simulink model "AircraftModel_6DoF_Chi"  (R2023b)
settings: Solver=VariableStepAuto  StartTime=0.0  StopTime=20  FixedStep=CNT_StepSize  RelTol=1e-3
values from neighbouring files (symbols this model uses):
  CNT_a = 6378137    [AircraftParameters.m]
  CNT_f = 0.003352810664747    (= 0.00335281066475)    [AircraftParameters.m]
  CNT_g = [0;0;9.81]    [AircraftParameters.m]
  CNT_m = 15975    [AircraftParameters.m]
  ControlLaws =     [ControlLaws.mat]
  Ixx = 102630    [AircraftParameters.m]
  Ixz = 14996    [AircraftParameters.m]
  Iyy = 274335    [AircraftParameters.m]
  Izz = 362250    [AircraftParameters.m]
undefined symbols (not defined in the file or in its folder): Actuators, Aerodynamics, ampl_p_cmd, ARI, beta_cmd, omega_p_cmd, Propulsion, TestSequence, TrimPoint
libraries: simulink x36, vrlib x4, slpidlib x1
(part 2 of 3)

== system AircraftModel_6DoF_Chi/Test Sequences/AoS Test Sequence ==
  Constant : Constant  Value=TrimPoint.States.Altbar
  Constant1 : Constant  Value=sqrt(TrimPoint.States.ubar^2+TrimPoint.States.vbar^2+TrimPoint.States.wbar^2)
  Constant2 : Constant  Value=TrimPoint.States.dabar
  Constant3 : Constant  Value=0
  Gust Generator : Subsystem  mask{gust_start=5, gust_duration=25, gust_amplitude=-30}
      mask prompts: gust_start "start time of the gust in sec"; gust_duration "gust duration in sec"; gust_amplitude "maximum gust speed in m/s"
      mask DialogControl ParameterGroupVar Prompt: gust characteristics
  Step : Step  Time=40  After=beta_cmd  SampleTime=0
  v_Wg : Outport
  u_Wg : Outport  Port=2
  alt_cmd : Outport  Port=3
  cmd_da : Outport  Port=4
  beta_cmd : Outport  Port=5
  V_A_cmd : Outport  Port=6
  wires:
  Constant3/1 -> u_Wg/1  "u_Wg"
  Constant2/1 -> cmd_da/1  "cmd_da"
  Constant1/1 -> V_A_cmd/1  "V_A_cmd"
  Step/1 -> beta_cmd/1  "beta_cmd"
  Constant/1 -> alt_cmd/1  "alt_cmd"
  Gust Generator/1(wind speed) -> v_Wg/1  "v_Wg"

== system AircraftModel_6DoF_Chi/Test Sequences/Bank Angle Test Sequence ==
  Constant : Constant  Value=TrimPoint.States.Altbar
  Constant1 : Constant  Value=sqrt(TrimPoint.States.ubar^2+TrimPoint.States.vbar^2+TrimPoint.States.wbar^2)
  Constant2 : Constant  Value=0
  Constant3 : Constant  Value=0
  Doublet Generator : Subsystem  mask(DoubletGenerator){timeon=5, pulsewidth=20, amplitude=deg2rad(55)}
      mask prompts: timeon "Time Start"; pulsewidth "Pulse Duration"
      mask help:
      | Doublet Generator.
      | Ouputs doublet of specificed amplitude and duration.
      |
      | If start/duration/amplitude parameters are vectors, then output is multichannel.
      mask Display: plot([.1 .3 .3001 .4 .4001 .5  .5001 .7],[0 0 1 1 -1 -1 0 0])
  Gust Generator : Subsystem  mask{gust_start=5, gust_duration=25, gust_amplitude=-30}
      mask prompts: gust_start "start time of the gust in sec"; gust_duration "gust duration in sec"; gust_amplitude "maximum gust speed in m/s"
      mask DialogControl ParameterGroupVar Prompt: gust characteristics
  v_Wg : Outport
  u_Wg : Outport  Port=2
  alt_cmd : Outport  Port=3
  Phi_cmd : Outport  Port=4
  beta_cmd : Outport  Port=5
  V_A_cmd : Outport  Port=6
  wires:
  Constant3/1 -> u_Wg/1  "u_Wg"
  Doublet Generator/1(Doublet) -> Phi_cmd/1  "Phi_cmd"
  Constant1/1 -> V_A_cmd/1  "V_A_cmd"
  Constant2/1 -> beta_cmd/1  "beta_cmd"
  Constant/1 -> alt_cmd/1  "alt_cmd"
  Gust Generator/1(wind speed) -> v_Wg/1  "v_Wg"

== system AircraftModel_6DoF_Chi/Test Sequences/Course Angle Test Sequence ==
  Constant : Constant  Value=TrimPoint.States.Altbar
  Constant1 : Constant  Value=sqrt(TrimPoint.States.ubar^2+TrimPoint.States.vbar^2+TrimPoint.States.wbar^2)
  Constant2 : Constant  Value=0
  Constant3 : Constant  Value=0
  Gust Generator : Subsystem  mask{gust_start=40, gust_duration=25, gust_amplitude=-30}
      mask prompts: gust_start "start time of the gust in sec"; gust_duration "gust duration in sec"; gust_amplitude "maximum gust speed in m/s"
      mask DialogControl ParameterGroupVar Prompt: gust characteristics
  Step1 : Step  Time=10  Before=TrimPoint.States.Psibar  After=deg2rad(350)  SampleTime=0
  v_Wg : Outport
  u_Wg : Outport  Port=2
  alt_cmd : Outport  Port=3
  Chi_cmd : Outport  Port=4
  beta_cmd : Outport  Port=5
  V_A_cmd : Outport  Port=6
  wires:
  Constant3/1 -> u_Wg/1  "u_Wg"
  Step1/1 -> Chi_cmd/1  "Chi_cmd"
  Constant1/1 -> V_A_cmd/1  "V_A_cmd"
  Constant2/1 -> beta_cmd/1  "beta_cmd"
  Constant/1 -> alt_cmd/1  "alt_cmd"
  Gust Generator/1(wind speed) -> v_Wg/1  "v_Wg"

== system AircraftModel_6DoF_Chi/Test Sequences/Default ==
  Constant : Constant  Value=TrimPoint.States.Altbar
  Constant1 : Constant  Value=sqrt(TrimPoint.States.ubar^2+TrimPoint.States.vbar^2+TrimPoint.States.wbar^2)
  Constant2 : Constant  Value=TrimPoint.States.dabar
  Constant3 : Constant  Value=0
  Constant4 : Constant  Value=TrimPoint.States.drbar
  Constant5 : Constant  Value=0
  v_Wg : Outport
  u_Wg : Outport  Port=2
  alt_cmd : Outport  Port=3
  cmd_da : Outport  Port=4
  cmd_dr : Outport  Port=5
  V_A_cmd : Outport  Port=6
  wires:
  Constant/1 -> alt_cmd/1  "alt_cmd"
  Constant1/1 -> V_A_cmd/1  "V_A_cmd"
  Constant2/1 -> cmd_da/1  "cmd_da"
  Constant4/1 -> cmd_dr/1  "cmd_dr"
  Constant5/1 -> v_Wg/1  "v_Wg"
  Constant3/1 -> u_Wg/1  "u_Wg"

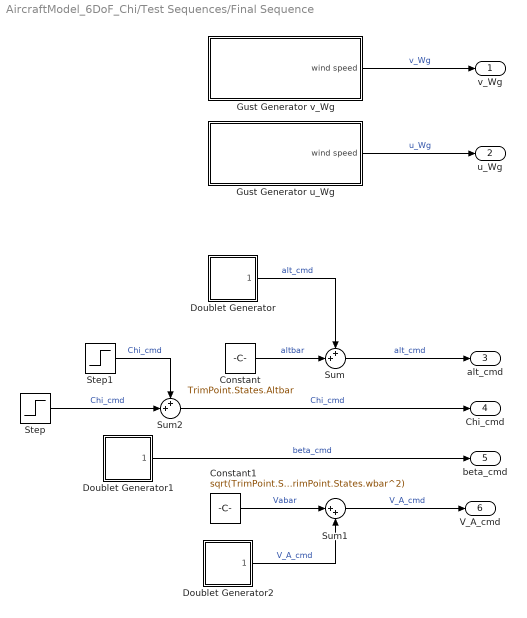
== system AircraftModel_6DoF_Chi/Test Sequences/Final Sequence ==
  Constant : Constant  Value=TrimPoint.States.Altbar
  Constant1 : Constant  Value=sqrt(TrimPoint.States.ubar^2+TrimPoint.States.vbar^2+TrimPoint.States.wbar^2)
  Doublet Generator : Subsystem  mask(DoubletGenerator){timeon=15, pulsewidth=40, amplitude=200}
      mask prompts: timeon "Time Start"; pulsewidth "Pulse Duration"
      mask help:
      | Doublet Generator.
      | Ouputs doublet of specificed amplitude and duration.
      |
      | If start/duration/amplitude parameters are vectors, then output is multichannel.
      mask Display: plot([.1 .3 .3001 .4 .4001 .5  .5001 .7],[0 0 1 1 -1 -1 0 0])
  Doublet Generator1 : Subsystem  mask(DoubletGenerator){timeon=60, pulsewidth=20, amplitude=deg2rad(3)}
      mask prompts: timeon "Time Start"; pulsewidth "Pulse Duration"
      mask help:
      | Doublet Generator.
      | Ouputs doublet of specificed amplitude and duration.
      |
      | If start/duration/amplitude parameters are vectors, then output is multichannel.
      mask Display: plot([.1 .3 .3001 .4 .4001 .5  .5001 .7],[0 0 1 1 -1 -1 0 0])
  Doublet Generator2 : Subsystem  mask(DoubletGenerator){timeon=10, pulsewidth=40, amplitude=-20}
      mask prompts: timeon "Time Start"; pulsewidth "Pulse Duration"
      mask help:
      | Doublet Generator.
      | Ouputs doublet of specificed amplitude and duration.
      |
      | If start/duration/amplitude parameters are vectors, then output is multichannel.
      mask Display: plot([.1 .3 .3001 .4 .4001 .5  .5001 .7],[0 0 1 1 -1 -1 0 0])
  Gust Generator u_Wg : Subsystem  mask{gust_start=60, gust_duration=15, gust_amplitude=-30}
      mask prompts: gust_start "start time of the gust in sec"; gust_duration "gust duration in sec"; gust_amplitude "maximum gust speed in m/s"
      mask DialogControl ParameterGroupVar Prompt: gust characteristics
  Gust Generator v_Wg : Subsystem  mask{gust_start=20, gust_duration=25, gust_amplitude=-30}
      mask prompts: gust_start "start time of the gust in sec"; gust_duration "gust duration in sec"; gust_amplitude "maximum gust speed in m/s"
      mask DialogControl ParameterGroupVar Prompt: gust characteristics
  Step : Step  Time=10  Before=TrimPoint.States.Psibar  After=deg2rad(10)  SampleTime=0
  Step1 : Step  Time=80  After=deg2rad(170)  SampleTime=0
  Sum : Sum  Inputs=++|
  Sum1 : Sum  Inputs=|++
  Sum2 : Sum  Inputs=++|
  v_Wg : Outport
  u_Wg : Outport  Port=2
  alt_cmd : Outport  Port=3
  Chi_cmd : Outport  Port=4
  beta_cmd : Outport  Port=5
  V_A_cmd : Outport  Port=6
  wires:
  Sum2/1 -> Chi_cmd/1  "Chi_cmd"
  Gust Generator u_Wg/1(wind speed) -> u_Wg/1  "u_Wg"
  Step1/1 -> Sum2/1  "Chi_cmd"
  Constant1/1 -> Sum1/1  "Vabar"
  Step/1 -> Sum2/2  "Chi_cmd"
  Doublet Generator/1(Doublet) -> Sum/1  "alt_cmd"
  Sum/1 -> alt_cmd/1  "alt_cmd"
  Gust Generator v_Wg/1(wind speed) -> v_Wg/1  "v_Wg"
  Doublet Generator2/1(Doublet) -> Sum1/2  "V_A_cmd"
  Constant/1 -> Sum/2  "altbar"
  Doublet Generator1/1(Doublet) -> beta_cmd/1  "beta_cmd"
  Sum1/1 -> V_A_cmd/1  "V_A_cmd"

== system AircraftModel_6DoF_Chi/Test Sequences/Roll Rate Test Sequence ==
  Constant : Constant  Value=TrimPoint.States.Altbar
  Constant1 : Constant  Value=sqrt(TrimPoint.States.ubar^2+TrimPoint.States.vbar^2+TrimPoint.States.wbar^2)
  Constant2 : Constant  Value=0
  Constant3 : Constant  Value=0
  Constant4 : Constant  Value=0
  Sine Wave1 : Sin  Amplitude=ampl_p_cmd  Frequency=omega_p_cmd  SampleTime=0
  v_Wg : Outport
  u_Wg : Outport  Port=2
  alt_cmd : Outport  Port=3
  p_cmd : Outport  Port=4
  beta_cmd : Outport  Port=5
  V_A_cmd : Outport  Port=6
  wires:
  Constant3/1 -> u_Wg/1  "u_Wg"
  Constant1/1 -> V_A_cmd/1  "V_A_cmd"
  Constant2/1 -> beta_cmd/1  "beta_cmd"
  Constant/1 -> alt_cmd/1  "alt_cmd"
  Constant4/1 -> v_Wg/1  "v_Wg"
  Sine Wave1/1 -> p_cmd/1  "p_cmd"

== system AircraftModel_6DoF_Chi/Test Sequences/SAS Test Sequence ==
  Constant : Constant  Value=TrimPoint.States.Altbar
  Constant1 : Constant  Value=sqrt(TrimPoint.States.ubar^2+TrimPoint.States.vbar^2+TrimPoint.States.wbar^2)
  Constant2 : Constant  Value=TrimPoint.States.dabar
  Constant3 : Constant  Value=0
  Gust Generator : Subsystem  mask{gust_start=5, gust_duration=25, gust_amplitude=-30}
      mask prompts: gust_start "start time of the gust in sec"; gust_duration "gust duration in sec"; gust_amplitude "maximum gust speed in m/s"
      mask DialogControl ParameterGroupVar Prompt: gust characteristics
  Step : Step  Time=40  After=deg2rad(5)  SampleTime=0
  v_Wg : Outport
  u_Wg : Outport  Port=2
  alt_cmd : Outport  Port=3
  cmd_da : Outport  Port=4
  cmd_dr : Outport  Port=5
  V_A_cmd : Outport  Port=6
  wires:
  Constant/1 -> alt_cmd/1  "alt_cmd"
  Constant1/1 -> V_A_cmd/1  "V_A_cmd"
  Constant2/1 -> cmd_da/1  "cmd_da"
  Step/1 -> cmd_dr/1  "cmd_dr"
  Gust Generator/1(wind speed) -> v_Wg/1  "v_Wg"
  Constant3/1 -> u_Wg/1  "u_Wg"

== system AircraftModel_6DoF_Chi/Equations of Motion/Calculation of Position_dot/ZeroOffset - cos (Lat) ==
  In : Inport
  Abs : Abs
  Constant : Constant  Value=tol  SampleTime=-1
  Non-zero Sign : Subsystem  mask(Non-zero sign){}
      mask help: Sign function outputs 1 for input greater than or equal to 0, and -1 otherwise.
  Product : Product  InputSameDT=on  SaturateOnIntegerOverflow=on  OutDataTypeStr=Inherit: Same as first input
  Switch : Switch  Threshold=tol
  Out : Outport
  wires:
  In/1 -> Switch/1, Non-zero Sign/1(In), Abs/1
  Abs/1 -> Switch/2
  Non-zero Sign/1(Out) -> Product/1
  Constant/1 -> Product/2
  Product/1 -> Switch/3
  Switch/1 -> Out/1

== system AircraftModel_6DoF_Chi/Flight Controls/Lateral Directional Control Laws/Aileron Rudder Interconnection ==
  cmd_da_in : Inport
  cmd_dr_in : Inport  Port=2
  ARI : Constant  Value=ARI
  Demux : Demux  Outputs=2
  Mux : Mux  Inputs=2
  Product : Product  Multiplication=Matrix(*)
  cmd_da_ARI : Outport
  cmd_dr_ARI : Outport  Port=2
  wires:
  cmd_da_in/1 -> Mux/1
  ARI/1 -> Product/1
  Demux/1 -> cmd_da_ARI/1
  Demux/2 -> cmd_dr_ARI/1
  Product/1 -> Demux/1
  cmd_dr_in/1 -> Mux/2
  Mux/1 -> Product/2

== system AircraftModel_6DoF_Chi/Flight Controls/Lateral Directional Control Laws/Bank Angle Control ==
  note: Proportional
      | Gain
  In1 : Inport
  Gain5 : Gain  Gain=ControlLaws.LatDirMot.BankAngle.Kp
  Saturation : Saturate  UpperLimit=12.5  LowerLimit=-12.5
  Out1 : Outport
  wires:
  Gain5/1 -> Saturation/1
  In1/1 -> Gain5/1
  Saturation/1 -> Out1/1

== system AircraftModel_6DoF_Chi/Flight Controls/Lateral Directional Control Laws/Course Angle Controller ==
  note: Proportional
      | Gain
  In1 : Inport
  Gain5 : Gain  Gain=ControlLaws.LatDirMot.Course.Kp
  Saturation : Saturate  UpperLimit=40  LowerLimit=-40
  Out1 : Outport
  wires:
  In1/1 -> Gain5/1
  Gain5/1 -> Saturation/1
  Saturation/1 -> Out1/1

== system AircraftModel_6DoF_Chi/Flight Controls/Lateral Directional Control Laws/Roll Rate Control ==
  note: Integrator Boost
  note: Lead/Lag Compensator
  note: Proportional
      | Gain
  note: Roll-Off Compensator
  In1 : Inport
  Input : Inport  Port=2
  Cond. Int. Anti Windup : Subsystem  mask(Integrator Anti-Windup){max_u=inf, min_u=-inf, negative_sign=off}
      mask prompts: max_u "Maximum control signal"; min_u "Minimum control signal"; negative_sign "Negative amplification in control law"
      mask help:
      | This block provides integration using the "conditional integration" anti-windup compensation.
      | It compares the sign of the error and the sign of the control signal and stops integration in case the error drives saturation.
      mask Help:
      | This block provides integration using the "conditional integration" anti-windup compensation. It stops or continues integration depending on the sign of the integrator input (control error) and the commanded control signal. Only if the input would further increase the already saturated integrator output, integration is stopped. This method is different from "integrator clamping" and and "integrator back calculation" and usually provides better recovery properties.
      | 
      | In a standard control architecture the inputs are as follows:
      | INPUT is the error signal r-y
      | RESET is a reset signal. The integrator state is reseted on either rising or falling edges
      | X0 is the initial condition for the integrator
      | U is the commanded control signal
      | 
      | For the anti-windup to work as intended, a saturation block must be placed on the ouput of the control command being fed to the associated actuator, which should include all control signal contributions (e.g. from proportional feedback and inner loops). U is the signal before this saturation.
      | 
      | The default logic assumes a plant with positive steady-state gain to be controlled. This translates to the following logic:
      | For commanded control signal u, saturation limits Umax and Umin, and error e,
      | If u is in bounds, do nothing
      | If u >= Umax AND e > 0, stop integrating
      | If u >= Umax AND e < 0, continue integrating
      | If u <= Umin AND e > 0, continue integrating
      | If u <= Umin AND e < 0, stop integrating
      | 
      | If a plant with negative steady-state gain is to be controlled (e.g. pitch), the windup logic may changed using the NEGATIVE SIGN option. (Note: If unsure check if the controller gains are negative. If yes, check the NEGATIVE SIGN option)
      | This then translates to the logic:
      | If u is in bounds, do nothing
      | If u >= Umax AND e < 0, stop integrating
      | If u >= Umax AND e > 0, continue integrating
      | If u <= Umin AND e < 0, continue integrating
      | If u <= Umin AND e > 0, stop integrating
  Gain3 : Gain  Gain=ControlLaws.LatDirMot.RollRate.Klz
  Gain4 : Gain  Gain=ControlLaws.LatDirMot.RollRate.Klp
  Gain5 : Gain  Gain=ControlLaws.LatDirMot.RollRate.Kp
  Gain6 : Gain  Gain=ControlLaws.LatDirMot.RollRate.Kr
  Gain7 : Gain  Gain=ControlLaws.LatDirMot.RollRate.Ki
  Integrator2 : Integrator  UpperSaturationLimit=max(Actuators.Limits.u_max_He)  LowerSaturationLimit=min(Actuators.Limits.u_max_He)  ContinuousStateAttributes='K'
  Integrator3 : Integrator  UpperSaturationLimit=max(Actuators.Limits.u_max_He)  LowerSaturationLimit=min(Actuators.Limits.u_max_He)  ContinuousStateAttributes='K'
  Integrator4 : Integrator  UpperSaturationLimit=max(Actuators.Limits.u_max_He)  LowerSaturationLimit=min(Actuators.Limits.u_max_He)  ContinuousStateAttributes='K'
  Integrator5 : Integrator  InitialCondition=TrimPoint.States.dabar  UpperSaturationLimit=max(Actuators.Limits.u_max_He)  LowerSaturationLimit=min(Actuators.Limits.u_max_He)  ContinuousStateAttributes='K'
  Saturation : Saturate  UpperLimit=max(Actuators.Limits.u_max_Hr)  LowerLimit=max(Actuators.Limits.u_max_Hr)
  Sum1 : Sum  Inputs=|++
  Sum3 : Sum  Inputs=|+-
  Sum6 : Sum  Inputs=|+-
  Sum7 : Sum  Inputs=|++
  cmd_da_in : Outport
  wires:
  Sum7/1 -> Saturation/1
  Integrator5/1 -> Sum7/1
  Gain5/1 -> Sum6/1
  Input/1 -> Cond. Int. Anti Windup/2(u)
  Gain7/1 -> Cond. Int. Anti Windup/1(in)
  Sum3/1 -> Gain7/1, Sum7/2, Gain4/1
  Gain6/1 -> Integrator4/1
  Cond. Int. Anti Windup/1(out) -> Integrator5/1
  Sum6/1 -> Gain6/1
  Saturation/1 -> cmd_da_in/1
  Gain4/1 -> Integrator3/1
  Integrator2/1 -> Sum1/1
  Sum1/1 -> Sum3/1
  Integrator3/1 -> Sum3/2
  Gain3/1 -> Integrator2/1
  Integrator4/1 -> Sum6/2, Sum1/2, Gain3/1
  In1/1 -> Gain5/1

== system AircraftModel_6DoF_Chi/Flight Controls/Lateral Directional Control Laws/Sideslip Angle Control ==
  note: Proportional
      | Gain
  note: Roll-Off Compensator
  note: Lead/Lag Compensator
  note: Integrator Boost
  In1 : Inport
  Input : Inport  Port=2
  Cond. Int. Anti Windup : Subsystem  mask(Integrator Anti-Windup){max_u=inf, min_u=-inf, negative_sign=off}
      mask prompts: max_u "Maximum control signal"; min_u "Minimum control signal"; negative_sign "Negative amplification in control law"
      mask help:
      | This block provides integration using the "conditional integration" anti-windup compensation.
      | It compares the sign of the error and the sign of the control signal and stops integration in case the error drives saturation.
      mask Help:
      | This block provides integration using the "conditional integration" anti-windup compensation. It stops or continues integration depending on the sign of the integrator input (control error) and the commanded control signal. Only if the input would further increase the already saturated integrator output, integration is stopped. This method is different from "integrator clamping" and and "integrator back calculation" and usually provides better recovery properties.
      | 
      | In a standard control architecture the inputs are as follows:
      | INPUT is the error signal r-y
      | RESET is a reset signal. The integrator state is reseted on either rising or falling edges
      | X0 is the initial condition for the integrator
      | U is the commanded control signal
      | 
      | For the anti-windup to work as intended, a saturation block must be placed on the ouput of the control command being fed to the associated actuator, which should include all control signal contributions (e.g. from proportional feedback and inner loops). U is the signal before this saturation.
      | 
      | The default logic assumes a plant with positive steady-state gain to be controlled. This translates to the following logic:
      | For commanded control signal u, saturation limits Umax and Umin, and error e,
      | If u is in bounds, do nothing
      | If u >= Umax AND e > 0, stop integrating
      | If u >= Umax AND e < 0, continue integrating
      | If u <= Umin AND e > 0, continue integrating
      | If u <= Umin AND e < 0, stop integrating
      | 
      | If a plant with negative steady-state gain is to be controlled (e.g. pitch), the windup logic may changed using the NEGATIVE SIGN option. (Note: If unsure check if the controller gains are negative. If yes, check the NEGATIVE SIGN option)
      | This then translates to the logic:
      | If u is in bounds, do nothing
      | If u >= Umax AND e < 0, stop integrating
      | If u >= Umax AND e > 0, continue integrating
      | If u <= Umin AND e < 0, continue integrating
      | If u <= Umin AND e > 0, stop integrating
  Gain3 : Gain  Gain=ControlLaws.LatDirMot.AoS.Klz
  Gain4 : Gain  Gain=ControlLaws.LatDirMot.AoS.Klp
  Gain5 : Gain  Gain=ControlLaws.LatDirMot.AoS.Kp
  Gain6 : Gain  Gain=ControlLaws.LatDirMot.AoS.Kr
  Gain7 : Gain  Gain=ControlLaws.LatDirMot.AoS.Ki
  Integrator2 : Integrator  UpperSaturationLimit=max(Actuators.Limits.u_max_He)  LowerSaturationLimit=min(Actuators.Limits.u_max_He)  ContinuousStateAttributes='K'
  Integrator3 : Integrator  UpperSaturationLimit=max(Actuators.Limits.u_max_He)  LowerSaturationLimit=min(Actuators.Limits.u_max_He)  ContinuousStateAttributes='K'
  Integrator4 : Integrator  UpperSaturationLimit=max(Actuators.Limits.u_max_He)  LowerSaturationLimit=min(Actuators.Limits.u_max_He)  ContinuousStateAttributes='K'
  Integrator5 : Integrator  InitialCondition=TrimPoint.States.drbar  UpperSaturationLimit=max(Actuators.Limits.u_max_He)  LowerSaturationLimit=min(Actuators.Limits.u_max_He)  ContinuousStateAttributes='K'
  Saturation : Saturate  UpperLimit=max(Actuators.Limits.u_max_Hr)  LowerLimit=max(Actuators.Limits.u_max_Hr)
  Sum1 : Sum  Inputs=|++
  Sum3 : Sum  Inputs=|+-
  Sum6 : Sum  Inputs=|+-
  Sum7 : Sum  Inputs=|++
  cmd_dr_in : Outport
  wires:
  In1/1 -> Gain5/1
  Saturation/1 -> cmd_dr_in/1
  Gain5/1 -> Sum6/1
  Sum6/1 -> Gain6/1
  Gain6/1 -> Integrator4/1
  Integrator4/1 -> Sum6/2, Sum1/2, Gain3/1
  Integrator3/1 -> Sum3/2
  Gain3/1 -> Integrator2/1
  Sum1/1 -> Sum3/1
  Gain4/1 -> Integrator3/1
  Integrator2/1 -> Sum1/1
  Sum7/1 -> Saturation/1
  Sum3/1 -> Gain7/1, Sum7/2, Gain4/1
  Integrator5/1 -> Sum7/1
  Gain7/1 -> Cond. Int. Anti Windup/1(in)
  Input/1 -> Cond. Int. Anti Windup/2(u)
  Cond. Int. Anti Windup/1(out) -> Integrator5/1

== system AircraftModel_6DoF_Chi/Flight Controls/Lateral Directional Control Laws/yaw damper ==
  note: LowPass Filter
  note: Proportional
      | Gain
  r : Inport
  Gain1 : Gain  Gain=ControlLaws.LatDirMot.SAS.omega_lp
  Gain5 : Gain  Gain=ControlLaws.LatDirMot.SAS.kr
  Integrator1 : Integrator  UpperSaturationLimit=max(Actuators.Limits.u_max_He)  LowerSaturationLimit=min(Actuators.Limits.u_max_He)  ContinuousStateAttributes='K'
  Sum2 : Sum  Inputs=|+-
  Washout Filter : Subsystem  mask{wb=ControlLaws.LatDirMot.SAS.omega_wo}
      mask prompts: wb "Filter Bandwidth"
      mask Display:
      | plot([0.35 0.5 0.65 ],[0.4 0.6 0.6 ]);
      | text(0.5,0.3,[num2str(wb) ' rad/s'],'horizontalAlignment', 'center');
      | text(0.67,0.6,['1'],'horizontalAlignment', 'left');
  dr : Outport
  wires:
  r/1 -> Washout Filter/1(Input)
  Sum2/1 -> Integrator1/1
  Gain1/1 -> Sum2/2
  Integrator1/1 -> Gain1/1, Gain5/1
  Washout Filter/1(Output) -> Sum2/1  "cmd_dr"
  Gain5/1 -> dr/1

== system AircraftModel_6DoF_Chi/Flight Controls/Longitudinal Control Laws/Subsystem ==
  Theta : Inport
  uf : Inport  Port=2
  wf : Inport  Port=3
  Cos : Trigonometry  Operator=cos
  Product : Product
  Product1 : Product
  Sin : Trigonometry
  Sum : Sum  Inputs=|+-
  hdot : Outport
  wires:
  Sum/1 -> hdot/1
  Product1/1 -> Sum/2
  Product/1 -> Sum/1
  Cos/1 -> Product1/1
  wf/1 -> Product1/2
  uf/1 -> Product/2
  Sin/1 -> Product/1
  Theta/1 -> Sin/1, Cos/1

== system AircraftModel_6DoF_Chi/Flight Controls/Longitudinal Control Laws/alt_control ==
  In1 : Inport
  Gain3 : Gain  Gain=ControlLaws.LonMot.Altitude.Klp
  Gain4 : Gain  Gain=10*ControlLaws.LonMot.Altitude.Klz
  Gain5 : Gain  Gain=ControlLaws.LonMot.Altitude.Kp
  Gain6 : Gain  Gain=ControlLaws.LonMot.Altitude.Kr
  Integrator2 : Integrator  UpperSaturationLimit=max(Actuators.Limits.u_max_He)  LowerSaturationLimit=min(Actuators.Limits.u_max_He)  ContinuousStateAttributes='Khdot'
  Integrator3 : Integrator  UpperSaturationLimit=max(Actuators.Limits.u_max_He)  LowerSaturationLimit=min(Actuators.Limits.u_max_He)  ContinuousStateAttributes='K'
  Integrator4 : Integrator  UpperSaturationLimit=max(Actuators.Limits.u_max_He)  LowerSaturationLimit=min(Actuators.Limits.u_max_He)  ContinuousStateAttributes='Khdot'
  Saturation2 : Saturate  UpperLimit=ControlLaws.Saturations.hdot(2)  LowerLimit=ControlLaws.Saturations.hdot(1)
  Sum1 : Sum  Inputs=|++
  Sum3 : Sum  Inputs=|+-
  Sum6 : Sum  Inputs=|+-
  Out1 : Outport
  wires:
  In1/1 -> Gain5/1
  Sum3/1 -> Sum6/1, Gain4/1
  Gain5/1 -> Gain3/1, Sum1/2
  Integrator4/1 -> Sum6/2, Saturation2/1
  Saturation2/1 -> Out1/1
  Integrator2/1 -> Sum1/1
  Sum1/1 -> Sum3/1
  Gain4/1 -> Integrator3/1
  Integrator3/1 -> Sum3/2
  Gain3/1 -> Integrator2/1
  Sum6/1 -> Gain6/1
  Gain6/1 -> Integrator4/1

== system AircraftModel_6DoF_Chi/Flight Controls/Longitudinal Control Laws/athrl_control ==
  In1 : Inport
  Gain2 : Gain  Gain=ControlLaws.LonMot.ATHR.Kr
  Gain3 : Gain  Gain=-ControlLaws.LonMot.ATHR.Kp
  Gain4 : Gain  Gain=ControlLaws.LonMot.ATHR.Klp
  Gain8 : Gain  Gain=ControlLaws.LonMot.ATHR.Klz
  Integrator1 : Integrator  UpperSaturationLimit=max(Actuators.Limits.u_max_He)  LowerSaturationLimit=min(Actuators.Limits.u_max_He)  ContinuousStateAttributes='K'
  Integrator2 : Integrator  UpperSaturationLimit=max(Actuators.Limits.u_max_He)  LowerSaturationLimit=min(Actuators.Limits.u_max_He)  ContinuousStateAttributes='K'
  Integrator3 : Integrator  UpperSaturationLimit=max(Actuators.Limits.u_max_He)  LowerSaturationLimit=min(Actuators.Limits.u_max_He)  ContinuousStateAttributes='K'
  Sum2 : Sum  Inputs=|+-
  Sum3 : Sum  Inputs=|++
  Sum4 : Sum  Inputs=|+-
  Out1 : Outport
  wires:
  Integrator2/1 -> Sum3/1
  Integrator3/1 -> Sum4/2
  Gain3/1 -> Gain4/1, Sum3/2
  In1/1 -> Gain3/1
  Sum3/1 -> Sum4/1
  Integrator1/1 -> Sum2/2, Out1/1
  Gain2/1 -> Integrator1/1
  Sum2/1 -> Gain2/1
  Gain4/1 -> Integrator2/1
  Gain8/1 -> Integrator3/1
  Sum4/1 -> Gain8/1, Sum2/1

== system AircraftModel_6DoF_Chi/Flight Controls/Longitudinal Control Laws/hdot_control ==
  In1 : Inport
  Gain3 : Gain  Gain=0.1*ControlLaws.LonMot.ClimbRate.Klp
  Gain4 : Gain  Gain=10*ControlLaws.LonMot.ClimbRate.Klz
  Gain5 : Gain  Gain="1.8  %ControlLaws.LonMot.ClimbRate.Kp"
  Gain6 : Gain  Gain=ControlLaws.LonMot.ClimbRate.Kr
  Integrator2 : Integrator  UpperSaturationLimit=max(Actuators.Limits.u_max_He)  LowerSaturationLimit=min(Actuators.Limits.u_max_He)  ContinuousStateAttributes='Khdot'
  Integrator3 : Integrator  UpperSaturationLimit=max(Actuators.Limits.u_max_He)  LowerSaturationLimit=min(Actuators.Limits.u_max_He)  ContinuousStateAttributes='K'
  Integrator4 : Integrator  UpperSaturationLimit=max(Actuators.Limits.u_max_He)  LowerSaturationLimit=min(Actuators.Limits.u_max_He)  ContinuousStateAttributes='Khdot'
  PID Controller : slpidlib/PID Controller  Controller=I  Form=Parallel  TimeDomain=Continuous-time  UseExternalTs=off  SampleTime=-1  IntegratorMethod=Forward Euler  FilterMethod=Forward Euler  ControllerParametersSource=internal  P=1.2  I=0.45  UseKiTs=off  D=1  N=100  UseFilter=on  TunerSelectOption=Transfer Function Based (PID Tuner App)  InitialConditionSource=internal  InitialConditionForIntegrator=0  InitialConditionForFilter=0  DifferentiatorICPrevScaledInput=0  ExternalReset=none  TrackingMode=off  Kt=1  LimitOutput=off  SatLimitsSource=internal  UpperSaturationLimit=inf  LowerSaturationLimit=-inf  LinearizeAsGain=on  AntiWindupMode=none  Kb=1  LimitIntegrator=off  UpperIntegratorSaturationLimit=inf  LowerIntegratorSaturationLimit=-inf  POutMin=[]  POutMax=[]  IOutMin=[]  IOutMax=[]  DOutMin=[]  DOutMax=[]  NOutMin=[]  NOutMax=[]  SumOutMin=[]  SumOutMax=[]  SaturationOutMin=[]  SaturationOutMax=[]  PParamMin=[]  PParamMax=[]  IParamMin=[]  IParamMax=[]  DParamMin=[]  DParamMax=[]  NParamMin=[]  NParamMax=[]  KbParamMin=[]  KbParamMax=[]  KtParamMin=[]  KtParamMax=[]  KbOutMin=[]  KbOutMax=[]  KtOutMin=[]  KtOutMax=[]  IntegratorOutMin=[]  IntegratorOutMax=[]  FilterOutMin=[]  FilterOutMax=[]  SumI1OutMin=[]  SumI1OutMax=[]  SumI2OutMin=[]  SumI2OutMax=[]  SumI3OutMin=[]  SumI3OutMax=[]  SumI4OutMin=[]  SumI4OutMax=[]  SumDOutMin=[]  SumDOutMax=[]  DifferentiatorOutMin=[]  DifferentiatorOutMax=[]  FilterDiffOutCoefMin=[]  FilterDiffOutCoefMax=[]  ReciprocalOutMin=[]  ReciprocalOutMax=[]  SumDenOutMin=[]  SumDenOutMax=[]  SumNumOutMin=[]  SumNumOutMax=[]  DivideOutMin=[]  DivideOutMax=[]  UdiffTsProdOutMin=[]  UdiffTsProdOutMax=[]  NTsProdOutMin=[]  NTsProdOutMax=[]  UintegralTsProdOutMin=[]  UintegralTsProdOutMax=[]  UngainTsProdOutMin=[]  UngainTsProdOutMax=[]  ClampingZeroOutDataTypeStr=Inherit: Inherit via back propagation  ClampingZeroOutMin=[]  ClampingZeroOutMax=[]  FilterDenConstantOutDataTypeStr=Inherit: Inherit via back propagation  FilterDenConstantOutMin=[]  FilterDenConstantOutMax=[]  PCopyOutDataTypeStr=Inherit: Inherit via back propagation  PCopyOutMin=[]  PCopyOutMax=[]  NCopyOutDataTypeStr=Inherit: Inherit via back propagation  NCopyOutMin=[]  NCopyOutMax=[]  IntegratorContinuousStateAttributes=''  IntegratorStateMustResolveToSignalObject=off  IntegratorRTWStateStorageClass=Auto  FilterContinuousStateAttributes=''  FilterStateMustResolveToSignalObject=off  FilterRTWStateStorageClass=Auto  ParallelPVariant=Disabled  IdealPVariant=Disabled  IVariant=InternalParameters  DVariant=Disabled  IntegratorVariant=Continuous  SatVariant=Disabled  AWVariant=Passthrough  PCopyVariant=Disabled  TRVariant=Disabled  FdbkBlocksVariant=Forward  IdealPFdbkVariant=Disabled  SatFdbkVariant=Disabled  DerivativeFilterVariant=Disabled  NVariant=Disabled  NCopyVariant=Disabled_SignalSpec  FilterICVariant=Disabled  IntegratorICVariant=InternalICs  ExternalResetVariant=Disabled  TRSumVariant=Passthrough  SumFdbkVariant=Disabled  SumVariant=Passthrough_I  TsampFilterVariant=InternalTs  TsampNgainVariant=Passthrough  TsampIntegralVariant=Disabled_SignalSpec  ExternalSaturationOutDataTypeStr=Inherit: Same as second input
  Saturation2 : Saturate  UpperLimit=ControlLaws.Saturations.nz(2)  LowerLimit=ControlLaws.Saturations.nz(1)
  Sum1 : Sum  Inputs=|++
  Sum3 : Sum  Inputs=|+-
  Sum6 : Sum  Inputs=|+-
  Out1 : Outport
  wires:
  PID Controller/1 -> Saturation2/1
  In1/1 -> Gain5/1
  Sum3/1 -> Sum6/1, Gain4/1
  Gain5/1 -> Gain3/1, Sum1/2
  Integrator4/1 -> Sum6/2, PID Controller/1
  Saturation2/1 -> Out1/1
  Integrator2/1 -> Sum1/1
  Sum1/1 -> Sum3/1
  Gain4/1 -> Integrator3/1
  Integrator3/1 -> Sum3/2
  Gain3/1 -> Integrator2/1
  Sum6/1 -> Gain6/1
  Gain6/1 -> Integrator4/1

== system AircraftModel_6DoF_Chi/Flight Controls/Longitudinal Control Laws/nz_control ==
  In1 : Inport
  Inport : Inport  Port=2
  Cond. Int. Anti Windup : Subsystem  mask(Integrator Anti-Windup){max_u=Actuators.Limits.u_max_He(2), min_u=Actuators.Limits.u_max_He(1), negative_sign=off}
      mask prompts: max_u "Maximum control signal"; min_u "Minimum control signal"; negative_sign "Negative amplification in control law"
      mask help:
      | This block provides integration using the "conditional integration" anti-windup compensation.
      | It compares the sign of the error and the sign of the control signal and stops integration in case the error drives saturation.
      mask Help:
      | This block provides integration using the "conditional integration" anti-windup compensation. It stops or continues integration depending on the sign of the integrator input (control error) and the commanded control signal. Only if the input would further increase the already saturated integrator output, integration is stopped. This method is different from "integrator clamping" and and "integrator back calculation" and usually provides better recovery properties.
      | 
      | In a standard control architecture the inputs are as follows:
      | INPUT is the error signal r-y
      | RESET is a reset signal. The integrator state is reseted on either rising or falling edges
      | X0 is the initial condition for the integrator
      | U is the commanded control signal
      | 
      | For the anti-windup to work as intended, a saturation block must be placed on the ouput of the control command being fed to the associated actuator, which should include all control signal contributions (e.g. from proportional feedback and inner loops). U is the signal before this saturation.
      | 
      | The default logic assumes a plant with positive steady-state gain to be controlled. This translates to the following logic:
      | For commanded control signal u, saturation limits Umax and Umin, and error e,
      | If u is in bounds, do nothing
      | If u >= Umax AND e > 0, stop integrating
      | If u >= Umax AND e < 0, continue integrating
      | If u <= Umin AND e > 0, continue integrating
      | If u <= Umin AND e < 0, stop integrating
      | 
      | If a plant with negative steady-state gain is to be controlled (e.g. pitch), the windup logic may changed using the NEGATIVE SIGN option. (Note: If unsure check if the controller gains are negative. If yes, check the NEGATIVE SIGN option)
      | This then translates to the logic:
      | If u is in bounds, do nothing
      | If u >= Umax AND e < 0, stop integrating
      | If u >= Umax AND e > 0, continue integrating
      | If u <= Umin AND e < 0, continue integrating
      | If u <= Umin AND e > 0, stop integrating
  Gain1 : Gain  Gain=ControlLaws.LonMot.LoadFactor.Kp
  Gain6 : Gain  Gain=ControlLaws.LonMot.LoadFactor.Kr
  Gain7 : Gain  Gain=ControlLaws.LonMot.LoadFactor.Ki
  Integrator4 : Integrator  UpperSaturationLimit=max(Actuators.Limits.u_max_He)  LowerSaturationLimit=min(Actuators.Limits.u_max_He)  ContinuousStateAttributes='Knz'
  Integrator5 : Integrator  UpperSaturationLimit=max(Actuators.Limits.u_max_He)  LowerSaturationLimit=min(Actuators.Limits.u_max_He)  ContinuousStateAttributes='Knz'
  Sum6 : Sum  Inputs=|+-
  Sum7 : Sum  Inputs=|++
  Out1 : Outport
  wires:
  Sum6/1 -> Gain6/1
  Integrator5/1 -> Sum7/1
  Inport/1 -> Cond. Int. Anti Windup/2(u)
  In1/1 -> Gain1/1
  Gain7/1 -> Cond. Int. Anti Windup/1(in)
  Integrator4/1 -> Gain7/1, Sum7/2, Sum6/2
  Cond. Int. Anti Windup/1(out) -> Integrator5/1
  Sum7/1 -> Out1/1
  Gain6/1 -> Integrator4/1
  Gain1/1 -> Sum6/1

== system AircraftModel_6DoF_Chi/Test Sequences/AoS Test Sequence/Gust Generator ==
  1-cos gust : Subsystem  TreatAsAtomicUnit=on
  Clock : Clock
  Compare To Constant : simulink/Logic and Bit Operations/Compare To Constant  relop=>=  const=gust_start  OutDataTypeStr=boolean
  Constant : Constant  Value=0
  Sum : Sum  Inputs=+-|
  Switch : Switch  Criteria=u2 > Threshold  Threshold=gust_start+gust_duration  SaturateOnIntegerOverflow=off  InputSameDT=off
  time freeze : Subsystem  TreatAsAtomicUnit=on
  wind speed : Outport
  wires:
  time freeze/1(out) -> Sum/2
  Constant/1 -> Switch/1
  Clock/1 -> time freeze/1(in), Compare To Constant/1, Sum/1, Switch/2
  Compare To Constant/1 -> 1-cos gust/Enable, time freeze/Trigger
  Sum/1 -> 1-cos gust/1(in)
  1-cos gust/1(wind) -> Switch/3
  Switch/1 -> wind speed/1

== system AircraftModel_6DoF_Chi/Test Sequences/Bank Angle Test Sequence/Doublet Generator ==
  Add : Sum  Inputs=+++
  DownStep : Step  Time=timeon+pulsewidth  After=-2  SampleTime=0
  Gain : Gain  Gain=amplitude
  UnStep : Step  Time=timeon+2*pulsewidth  SampleTime=0
  UpStep : Step  Time=timeon  SampleTime=0
  Doublet : Outport
  wires:
  UpStep/1 -> Add/1
  DownStep/1 -> Add/2
  UnStep/1 -> Add/3
  Add/1 -> Gain/1
  Gain/1 -> Doublet/1

== system AircraftModel_6DoF_Chi/Test Sequences/Bank Angle Test Sequence/Gust Generator ==
  1-cos gust : Subsystem  TreatAsAtomicUnit=on
  Clock : Clock
  Compare To Constant : simulink/Logic and Bit Operations/Compare To Constant  relop=>=  const=gust_start  OutDataTypeStr=boolean
  Constant : Constant  Value=0
  Sum : Sum  Inputs=+-|
  Switch : Switch  Criteria=u2 > Threshold  Threshold=gust_start+gust_duration  SaturateOnIntegerOverflow=off  InputSameDT=off
  time freeze : Subsystem  TreatAsAtomicUnit=on
  wind speed : Outport
  wires:
  time freeze/1(out) -> Sum/2
  Constant/1 -> Switch/1
  Clock/1 -> time freeze/1(in), Compare To Constant/1, Sum/1, Switch/2
  Compare To Constant/1 -> 1-cos gust/Enable, time freeze/Trigger
  Sum/1 -> 1-cos gust/1(in)
  1-cos gust/1(wind) -> Switch/3
  Switch/1 -> wind speed/1

== system AircraftModel_6DoF_Chi/Test Sequences/Course Angle Test Sequence/Gust Generator ==
  1-cos gust : Subsystem  TreatAsAtomicUnit=on
  Clock : Clock
  Compare To Constant : simulink/Logic and Bit Operations/Compare To Constant  relop=>=  const=gust_start  OutDataTypeStr=boolean
  Constant : Constant  Value=0
  Sum : Sum  Inputs=+-|
  Switch : Switch  Criteria=u2 > Threshold  Threshold=gust_start+gust_duration  SaturateOnIntegerOverflow=off  InputSameDT=off
  time freeze : Subsystem  TreatAsAtomicUnit=on
  wind speed : Outport
  wires:
  time freeze/1(out) -> Sum/2
  Constant/1 -> Switch/1
  Clock/1 -> time freeze/1(in), Compare To Constant/1, Sum/1, Switch/2
  Compare To Constant/1 -> 1-cos gust/Enable, time freeze/Trigger
  Sum/1 -> 1-cos gust/1(in)
  1-cos gust/1(wind) -> Switch/3
  Switch/1 -> wind speed/1

== system AircraftModel_6DoF_Chi/Test Sequences/Final Sequence/Doublet Generator ==
  Add : Sum  Inputs=+++
  DownStep : Step  Time=timeon+pulsewidth  After=-2  SampleTime=0
  Gain : Gain  Gain=amplitude
  UnStep : Step  Time=timeon+2*pulsewidth  SampleTime=0
  UpStep : Step  Time=timeon  SampleTime=0
  Doublet : Outport
  wires:
  UpStep/1 -> Add/1
  DownStep/1 -> Add/2
  UnStep/1 -> Add/3
  Add/1 -> Gain/1
  Gain/1 -> Doublet/1

== system AircraftModel_6DoF_Chi/Test Sequences/Final Sequence/Doublet Generator1 ==
  Add : Sum  Inputs=+++
  DownStep : Step  Time=timeon+pulsewidth  After=-2  SampleTime=0
  Gain : Gain  Gain=amplitude
  UnStep : Step  Time=timeon+2*pulsewidth  SampleTime=0
  UpStep : Step  Time=timeon  SampleTime=0
  Doublet : Outport
  wires:
  UpStep/1 -> Add/1
  DownStep/1 -> Add/2
  UnStep/1 -> Add/3
  Add/1 -> Gain/1
  Gain/1 -> Doublet/1

== system AircraftModel_6DoF_Chi/Test Sequences/Final Sequence/Doublet Generator2 ==
  Add : Sum  Inputs=+++
  DownStep : Step  Time=timeon+pulsewidth  After=-2  SampleTime=0
  Gain : Gain  Gain=amplitude
  UnStep : Step  Time=timeon+2*pulsewidth  SampleTime=0
  UpStep : Step  Time=timeon  SampleTime=0
  Doublet : Outport
  wires:
  UpStep/1 -> Add/1
  DownStep/1 -> Add/2
  UnStep/1 -> Add/3
  Add/1 -> Gain/1
  Gain/1 -> Doublet/1

== system AircraftModel_6DoF_Chi/Test Sequences/Final Sequence/Gust Generator u_Wg ==
  1-cos gust : Subsystem  TreatAsAtomicUnit=on
  Clock : Clock
  Compare To Constant : simulink/Logic and Bit Operations/Compare To Constant  relop=>=  const=gust_start  OutDataTypeStr=boolean
  Constant : Constant  Value=0
  Sum : Sum  Inputs=+-|
  Switch : Switch  Criteria=u2 > Threshold  Threshold=gust_start+gust_duration  SaturateOnIntegerOverflow=off  InputSameDT=off
  time freeze : Subsystem  TreatAsAtomicUnit=on
  wind speed : Outport
  wires:
  time freeze/1(out) -> Sum/2
  Constant/1 -> Switch/1
  Clock/1 -> time freeze/1(in), Compare To Constant/1, Sum/1, Switch/2
  Compare To Constant/1 -> 1-cos gust/Enable, time freeze/Trigger
  Sum/1 -> 1-cos gust/1(in)
  1-cos gust/1(wind) -> Switch/3
  Switch/1 -> wind speed/1

== system AircraftModel_6DoF_Chi/Test Sequences/Final Sequence/Gust Generator v_Wg ==
  1-cos gust : Subsystem  TreatAsAtomicUnit=on
  Clock : Clock
  Compare To Constant : simulink/Logic and Bit Operations/Compare To Constant  relop=>=  const=gust_start  OutDataTypeStr=boolean
  Constant : Constant  Value=0
  Sum : Sum  Inputs=+-|
  Switch : Switch  Criteria=u2 > Threshold  Threshold=gust_start+gust_duration  SaturateOnIntegerOverflow=off  InputSameDT=off
  time freeze : Subsystem  TreatAsAtomicUnit=on
  wind speed : Outport
  wires:
  time freeze/1(out) -> Sum/2
  Constant/1 -> Switch/1
  Clock/1 -> time freeze/1(in), Compare To Constant/1, Sum/1, Switch/2
  Compare To Constant/1 -> 1-cos gust/Enable, time freeze/Trigger
  Sum/1 -> 1-cos gust/1(in)
  1-cos gust/1(wind) -> Switch/3
  Switch/1 -> wind speed/1

== system AircraftModel_6DoF_Chi/Test Sequences/SAS Test Sequence/Gust Generator ==
  1-cos gust : Subsystem  TreatAsAtomicUnit=on
  Clock : Clock
  Compare To Constant : simulink/Logic and Bit Operations/Compare To Constant  relop=>=  const=gust_start  OutDataTypeStr=boolean
  Constant : Constant  Value=0
  Sum : Sum  Inputs=+-|
  Switch : Switch  Criteria=u2 > Threshold  Threshold=gust_start+gust_duration  SaturateOnIntegerOverflow=off  InputSameDT=off
  time freeze : Subsystem  TreatAsAtomicUnit=on
  wind speed : Outport
  wires:
  time freeze/1(out) -> Sum/2
  Constant/1 -> Switch/1
  Clock/1 -> time freeze/1(in), Compare To Constant/1, Sum/1, Switch/2
  Compare To Constant/1 -> 1-cos gust/Enable, time freeze/Trigger
  Sum/1 -> 1-cos gust/1(in)
  1-cos gust/1(wind) -> Switch/3
  Switch/1 -> wind speed/1

== system AircraftModel_6DoF_Chi/Equations of Motion/Calculation of Position_dot/ZeroOffset - cos (Lat)/Non-zero Sign ==
  In : Inport
  One : Constant  SampleTime=-1
  Relational Operator : RelationalOperator  Operator===
  Sign : Signum
  Switch : Switch  Threshold=1
  Zero : Constant  Value=0  SampleTime=-1
  Out : Outport
  wires:
  Zero/1 -> Relational Operator/2
  In/1 -> Relational Operator/1, Sign/1
  Relational Operator/1 -> Switch/2
  One/1 -> Switch/1
  Sign/1 -> Switch/3
  Switch/1 -> Out/1

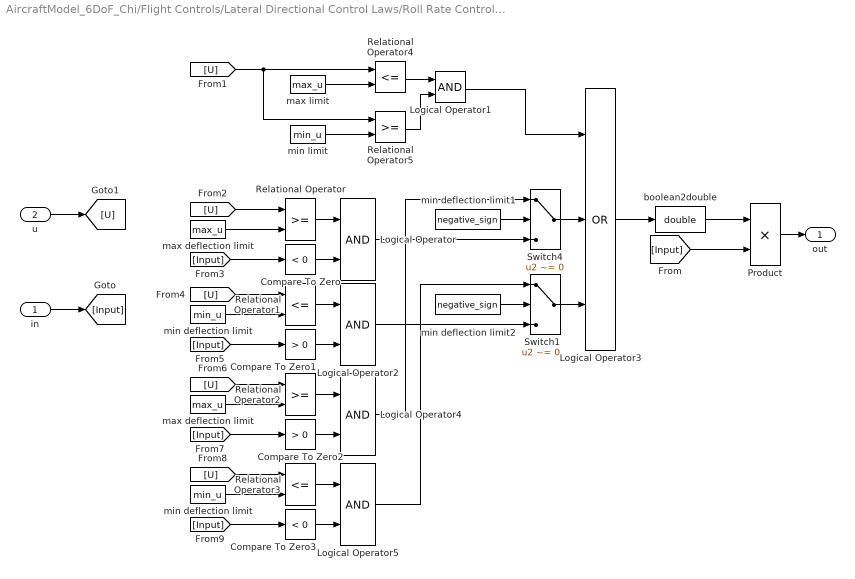
== system AircraftModel_6DoF_Chi/Flight Controls/Lateral Directional Control Laws/Roll Rate Control/Cond. Int. Anti Windup ==
  in : Inport
  u : Inport  Port=2
  Compare To Zero : simulink/Logic and Bit Operations/Compare To Zero  relop=<  OutDataTypeStr=uint8
  Compare To Zero1 : simulink/Logic and Bit Operations/Compare To Zero  relop=>  OutDataTypeStr=uint8
  Compare To Zero2 : simulink/Logic and Bit Operations/Compare To Zero  relop=>  OutDataTypeStr=uint8
  Compare To Zero3 : simulink/Logic and Bit Operations/Compare To Zero  relop=<  OutDataTypeStr=uint8
  Logical Operator{,1..2,4..5} (5 alike) : Logic  AllPortsSameDT=off  OutDataTypeStr=boolean
  Logical Operator3 : Logic  Operator=OR  Inputs=3  AllPortsSameDT=off  OutDataTypeStr=boolean
  Product : Product
  Relational Operator : RelationalOperator  OutDataTypeStr=boolean  InputSameDT=off
  Relational Operator1 : RelationalOperator  Operator=<=  OutDataTypeStr=boolean  InputSameDT=off
  Relational Operator2 : RelationalOperator  OutDataTypeStr=boolean  InputSameDT=off
  Relational Operator3 : RelationalOperator  Operator=<=  OutDataTypeStr=boolean  InputSameDT=off
  Relational Operator4 : RelationalOperator  Operator=<=  OutDataTypeStr=boolean  InputSameDT=off
  Relational Operator5 : RelationalOperator  OutDataTypeStr=boolean  InputSameDT=off
  Switch1 : Switch  Criteria=u2 ~= 0  SaturateOnIntegerOverflow=off  InputSameDT=off
  Switch4 : Switch  Criteria=u2 ~= 0  SaturateOnIntegerOverflow=off  InputSameDT=off
  boolean2double : DataTypeConversion  OutDataTypeStr=double  SaturateOnIntegerOverflow=off  RndMeth=Floor
  max deflection limit : Constant  Value=max_u  SampleTime=-1
  "max deflection limit " : Constant  Value=max_u  SampleTime=-1
  max limit : Constant  Value=max_u  SampleTime=-1
  min deflection limit : Constant  Value=min_u  SampleTime=-1
  "min deflection limit " : Constant  Value=min_u  SampleTime=-1
  min deflection limit1 : Constant  Value=negative_sign  SampleTime=-1
  min deflection limit2 : Constant  Value=negative_sign  SampleTime=-1
  min limit : Constant  Value=min_u  SampleTime=-1
  out : Outport
  wires:
  Product/1 -> out/1
  Logical Operator3/1 -> boolean2double/1
  boolean2double/1 -> Product/1
  [Input] -> Product/2
  [Input] -> Compare To Zero3/1
  [U] -> Relational Operator3/1
  [Input] -> Compare To Zero2/1
  [U] -> Relational Operator2/1
  [Input] -> Compare To Zero1/1
  [U] -> Relational Operator1/1
  [Input] -> Compare To Zero/1
  [U] -> Relational Operator/1
  [U] -> Relational Operator4/1, Relational Operator5/1
  u/1 -> [U]
  in/1 -> [Input]
  min limit/1 -> Relational Operator5/2
  Relational Operator5/1 -> Logical Operator1/2
  Relational Operator4/1 -> Logical Operator1/1
  max limit/1 -> Relational Operator4/2
  Logical Operator5/1 -> Switch1/1
  Logical Operator4/1 -> Switch4/1
  Logical Operator2/1 -> Switch1/3
  Logical Operator/1 -> Switch4/3
  min deflection limit1/1 -> Switch4/2
  Switch1/1 -> Logical Operator3/3
  min deflection limit2/1 -> Switch1/2
  max deflection limit/1 -> Relational Operator/2
  Compare To Zero/1 -> Logical Operator/2
  Relational Operator/1 -> Logical Operator/1
  Compare To Zero1/1 -> Logical Operator2/2
  Relational Operator1/1 -> Logical Operator2/1
  min deflection limit/1 -> Relational Operator1/2
  Switch4/1 -> Logical Operator3/2
  Logical Operator1/1 -> Logical Operator3/1
  Compare To Zero2/1 -> Logical Operator4/2
  Relational Operator2/1 -> Logical Operator4/1
  Compare To Zero3/1 -> Logical Operator5/2
  Relational Operator3/1 -> Logical Operator5/1
  "min deflection limit "/1 -> Relational Operator3/2
  "max deflection limit "/1 -> Relational Operator2/2

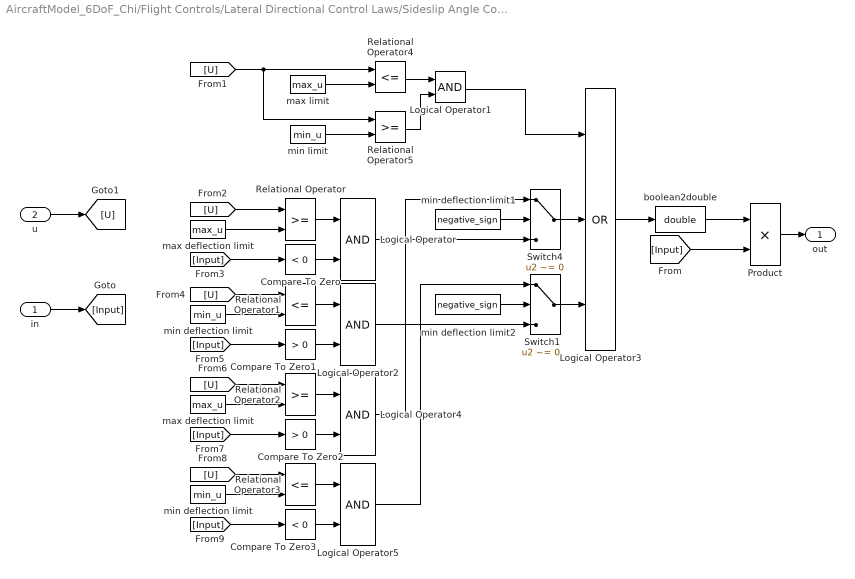
== system AircraftModel_6DoF_Chi/Flight Controls/Lateral Directional Control Laws/Sideslip Angle Control/Cond. Int. Anti Windup ==
  in : Inport
  u : Inport  Port=2
  Compare To Zero : simulink/Logic and Bit Operations/Compare To Zero  relop=<  OutDataTypeStr=uint8
  Compare To Zero1 : simulink/Logic and Bit Operations/Compare To Zero  relop=>  OutDataTypeStr=uint8
  Compare To Zero2 : simulink/Logic and Bit Operations/Compare To Zero  relop=>  OutDataTypeStr=uint8
  Compare To Zero3 : simulink/Logic and Bit Operations/Compare To Zero  relop=<  OutDataTypeStr=uint8
  Logical Operator{,1..2,4..5} (5 alike) : Logic  AllPortsSameDT=off  OutDataTypeStr=boolean
  Logical Operator3 : Logic  Operator=OR  Inputs=3  AllPortsSameDT=off  OutDataTypeStr=boolean
  Product : Product
  Relational Operator : RelationalOperator  OutDataTypeStr=boolean  InputSameDT=off
  Relational Operator1 : RelationalOperator  Operator=<=  OutDataTypeStr=boolean  InputSameDT=off
  Relational Operator2 : RelationalOperator  OutDataTypeStr=boolean  InputSameDT=off
  Relational Operator3 : RelationalOperator  Operator=<=  OutDataTypeStr=boolean  InputSameDT=off
  Relational Operator4 : RelationalOperator  Operator=<=  OutDataTypeStr=boolean  InputSameDT=off
  Relational Operator5 : RelationalOperator  OutDataTypeStr=boolean  InputSameDT=off
  Switch1 : Switch  Criteria=u2 ~= 0  SaturateOnIntegerOverflow=off  InputSameDT=off
  Switch4 : Switch  Criteria=u2 ~= 0  SaturateOnIntegerOverflow=off  InputSameDT=off
  boolean2double : DataTypeConversion  OutDataTypeStr=double  SaturateOnIntegerOverflow=off  RndMeth=Floor
  max deflection limit : Constant  Value=max_u  SampleTime=-1
  "max deflection limit " : Constant  Value=max_u  SampleTime=-1
  max limit : Constant  Value=max_u  SampleTime=-1
  min deflection limit : Constant  Value=min_u  SampleTime=-1
  "min deflection limit " : Constant  Value=min_u  SampleTime=-1
  min deflection limit1 : Constant  Value=negative_sign  SampleTime=-1
  min deflection limit2 : Constant  Value=negative_sign  SampleTime=-1
  min limit : Constant  Value=min_u  SampleTime=-1
  out : Outport
  wires:
  Product/1 -> out/1
  Logical Operator3/1 -> boolean2double/1
  boolean2double/1 -> Product/1
  [Input] -> Product/2
  [Input] -> Compare To Zero3/1
  [U] -> Relational Operator3/1
  [Input] -> Compare To Zero2/1
  [U] -> Relational Operator2/1
  [Input] -> Compare To Zero1/1
  [U] -> Relational Operator1/1
  [Input] -> Compare To Zero/1
  [U] -> Relational Operator/1
  [U] -> Relational Operator4/1, Relational Operator5/1
  u/1 -> [U]
  in/1 -> [Input]
  min limit/1 -> Relational Operator5/2
  Relational Operator5/1 -> Logical Operator1/2
  Relational Operator4/1 -> Logical Operator1/1
  max limit/1 -> Relational Operator4/2
  Logical Operator5/1 -> Switch1/1
  Logical Operator4/1 -> Switch4/1
  Logical Operator2/1 -> Switch1/3
  Logical Operator/1 -> Switch4/3
  min deflection limit1/1 -> Switch4/2
  Switch1/1 -> Logical Operator3/3
  min deflection limit2/1 -> Switch1/2
  max deflection limit/1 -> Relational Operator/2
  Compare To Zero/1 -> Logical Operator/2
  Relational Operator/1 -> Logical Operator/1
  Compare To Zero1/1 -> Logical Operator2/2
  Relational Operator1/1 -> Logical Operator2/1
  min deflection limit/1 -> Relational Operator1/2
  Switch4/1 -> Logical Operator3/2
  Logical Operator1/1 -> Logical Operator3/1
  Compare To Zero2/1 -> Logical Operator4/2
  Relational Operator2/1 -> Logical Operator4/1
  Compare To Zero3/1 -> Logical Operator5/2
  Relational Operator3/1 -> Logical Operator5/1
  "min deflection limit "/1 -> Relational Operator3/2
  "max deflection limit "/1 -> Relational Operator2/2

== system AircraftModel_6DoF_Chi/Flight Controls/Lateral Directional Control Laws/yaw damper/Washout Filter ==
  Input : Inport
  Gain : Gain  Gain=wb
  Gain1 : Gain  Gain=wb
  Integrator : Integrator  ContinuousStateAttributes='K_wo'
  Sum3 : Sum  Inputs=++|
  Sum5 : Sum  Inputs=|--
  Output : Outport
  wires:
  Gain/1 -> Sum5/2
  Integrator/1 -> Gain/1, Sum3/2
  Input/1 -> Gain1/1, Sum3/1
  Sum5/1 -> Integrator/1
  Gain1/1 -> Sum5/1
  Sum3/1 -> Output/1
